simulink model "axi_stream_sobel_filter"  (R2020a)
settings: Solver=VariableStepAuto  StartTime=0.0  StopTime=(height*width)/fs + (width*6)/fs + 128/fs  RelTol=1e-3
PreLoadFcn:
  | clear all;
  | 
  | fs = 100e6;
PostLoadFcn:
  | ratio = 1/6;
  | set(0,'units','pixels');
  | pixels = get(0,'screensize');
  | point1 = round(pixels(3)*ratio);
  | point2 = round(pixels(4)*ratio);
  | point3 = pixels(3)-round(pixels(3)*ratio);
  | point4 = pixels(4)-round(pixels(4)*ratio);
  | h = get_param(gcs,'handle');
  | set_param(h,'location',[point1 point2 point3 point4]);
  | pause(0.2);
  | set_param(h,'Zoomfactor','fit to view');
  | 
  | clear ratio pixels point1 point2 point3 point4 h
  | 
  | % https://uk.mathworks.com/matlabcentral/answers/358413-open-simulink-model-with-set-window-size-and-position
InitFcn:
  | height = str2num(get_param([bdroot, '/Image Properties'], 'height'));
  | width = str2num(get_param([bdroot, '/Image Properties'], 'width'));
  | I = imresize(eval(get_param([bdroot, '/Image Properties'], 'image')), [(height) (width)]);
  | I = padarray(I, [1 1], 'replicate');
  | bufferOut = uint32(double(I(:,:,1))*2^16 + double(I(:,:,3))*2^8 + double(I(:,:,2)));
  | bufferOut = reshape(bufferOut', [width+2, height+2]);
  | bufferOut = bufferOut(:);
StopFcn:
  | imtool(I);
  | imtool(uint8(reshape(bufferIn, [width, height])'));
undefined symbols (not defined in the file): AXI4, Lite
libraries: xbsIndex_r4 x131, hdlsllib x3, dspsrcs4 x2, simulink x1
(part 2 of 2)

== system axi_stream_sobel_filter/DUT/Algorithm/Sobel Edge Filter/Thresholding ==
  Threshold : Inport
  Gmag : Inport  Port=2
  Constant : xbsIndex_r4/Constant  const=255  gui_display_data_type=Fixed-point  arith_type=Unsigned  n_bits=8  bin_pt=0  preci_type=Single  exp_width=8  frac_width=24  explicit_period=on  period=1/100e6  equ=P=C  opselect=C  inp2=PCIN>>17  opr=+  inp1=P  carry=CIN  dbl_ovrd=off  block_type=constant
  Constant1 : xbsIndex_r4/Constant  const=0  gui_display_data_type=Fixed-point  arith_type=Unsigned  n_bits=8  bin_pt=0  preci_type=Single  exp_width=8  frac_width=24  explicit_period=on  period=1/100e6  equ=P=C  opselect=C  inp2=PCIN>>17  opr=+  inp1=P  carry=CIN  dbl_ovrd=off  block_type=constant
  Mux : xbsIndex_r4/Mux  inputs=2  en=off  latency=1  precision=Full  arith_type=Unsigned  n_bits=16  bin_pt=14  quantization=Truncate  overflow=Wrap  dbl_ovrd=off  block_type=mux
  Relational : xbsIndex_r4/Relational  mode=a>=b  op_type=Bool  en=off  latency=0  dbl_ovrd=off  block_type=relational
  Edge : Outport  VectorParamsAs1DForOutWhenUnconnected=off
  wires:
  Threshold/1 -> Relational/2
  Relational/1 -> Mux/1
  Constant/1 -> Mux/3
  Constant1/1 -> Mux/2
  Gmag/1 -> Relational/1
  Mux/1 -> Edge/1

== system axi_stream_sobel_filter/DUT/Algorithm/Sobel Edge Filter/Filter Function/Gx Operation ==
  w00 : Inport
  w02 : Inport  Port=2
  w10 : Inport  Port=3
  w12 : Inport  Port=4
  w20 : Inport  Port=5
  w22 : Inport  Port=6
  AddSub : xbsIndex_r4/AddSub  mode=Subtraction  use_carryin=off  use_carryout=off  en=off  latency=1  precision=Full  arith_type=Unsigned  n_bits=16  bin_pt=14  quantization=Truncate  overflow=Wrap  use_behavioral_HDL=off  hw_selection=Fabric  pipelined=off  dbl_ovrd=off  block_type=addsub
  AddSub1 : xbsIndex_r4/AddSub  mode=Subtraction  use_carryin=off  use_carryout=off  en=off  latency=1  precision=Full  arith_type=Unsigned  n_bits=16  bin_pt=14  quantization=Truncate  overflow=Wrap  use_behavioral_HDL=off  hw_selection=Fabric  pipelined=off  dbl_ovrd=off  block_type=addsub
  AddSub2 : xbsIndex_r4/AddSub  mode=Subtraction  use_carryin=off  use_carryout=off  en=off  latency=1  precision=Full  arith_type=Unsigned  n_bits=16  bin_pt=14  quantization=Truncate  overflow=Wrap  use_behavioral_HDL=off  hw_selection=Fabric  pipelined=off  dbl_ovrd=off  block_type=addsub
  AddSub3 : xbsIndex_r4/AddSub  mode=Addition  use_carryin=off  use_carryout=off  en=off  latency=1  precision=Full  arith_type=Unsigned  n_bits=16  bin_pt=14  quantization=Truncate  overflow=Wrap  use_behavioral_HDL=off  hw_selection=Fabric  pipelined=off  dbl_ovrd=off  block_type=addsub
  AddSub4 : xbsIndex_r4/AddSub  mode=Addition  use_carryin=off  use_carryout=off  en=off  latency=1  precision=Full  arith_type=Unsigned  n_bits=16  bin_pt=14  quantization=Truncate  overflow=Wrap  use_behavioral_HDL=off  hw_selection=Fabric  pipelined=off  dbl_ovrd=off  block_type=addsub
  CMult : xbsIndex_r4/CMult  const=2  gui_display_data_type=Fixed-point  const_n_bits=2  const_bin_pt=0  float_type=Single  exp_bits=8  fraction_bits=24  en=off  latency=1  precision=Full  arith_type="Signed  (2's comp)"  n_bits=16  bin_pt=14  quantization=Truncate  overflow=Wrap  use_behavioral_HDL=off  mem_type=Distributed RAM  pipeline=off  dbl_ovrd=off  block_type=cmult
  CMult1 : xbsIndex_r4/CMult  const=2  gui_display_data_type=Fixed-point  const_n_bits=2  const_bin_pt=0  float_type=Single  exp_bits=8  fraction_bits=24  en=off  latency=1  precision=Full  arith_type="Signed  (2's comp)"  n_bits=16  bin_pt=14  quantization=Truncate  overflow=Wrap  use_behavioral_HDL=off  mem_type=Distributed RAM  pipeline=off  dbl_ovrd=off  block_type=cmult
  Gx : Outport  VectorParamsAs1DForOutWhenUnconnected=off
  wires:
  AddSub4/1 -> Gx/1
  AddSub1/1 -> AddSub4/2
  AddSub3/1 -> AddSub4/1
  AddSub2/1 -> AddSub3/2
  w20/1 -> AddSub2/2
  w22/1 -> AddSub2/1
  AddSub/1 -> AddSub3/1
  CMult/1 -> AddSub1/2
  CMult1/1 -> AddSub1/1
  w12/1 -> CMult1/1
  w10/1 -> CMult/1
  w00/1 -> AddSub/2
  w02/1 -> AddSub/1

== system axi_stream_sobel_filter/DUT/Algorithm/Sobel Edge Filter/Filter Function/Gy Operation ==
  w00 : Inport
  w01 : Inport  Port=2
  w02 : Inport  Port=3
  w20 : Inport  Port=4
  w21 : Inport  Port=5
  w22 : Inport  Port=6
  AddSub : xbsIndex_r4/AddSub  mode=Subtraction  use_carryin=off  use_carryout=off  en=off  latency=1  precision=Full  arith_type=Unsigned  n_bits=16  bin_pt=14  quantization=Truncate  overflow=Wrap  use_behavioral_HDL=off  hw_selection=Fabric  pipelined=off  dbl_ovrd=off  block_type=addsub
  AddSub1 : xbsIndex_r4/AddSub  mode=Subtraction  use_carryin=off  use_carryout=off  en=off  latency=1  precision=Full  arith_type=Unsigned  n_bits=16  bin_pt=14  quantization=Truncate  overflow=Wrap  use_behavioral_HDL=off  hw_selection=Fabric  pipelined=off  dbl_ovrd=off  block_type=addsub
  AddSub2 : xbsIndex_r4/AddSub  mode=Subtraction  use_carryin=off  use_carryout=off  en=off  latency=1  precision=Full  arith_type=Unsigned  n_bits=16  bin_pt=14  quantization=Truncate  overflow=Wrap  use_behavioral_HDL=off  hw_selection=Fabric  pipelined=off  dbl_ovrd=off  block_type=addsub
  AddSub3 : xbsIndex_r4/AddSub  mode=Addition  use_carryin=off  use_carryout=off  en=off  latency=1  precision=Full  arith_type=Unsigned  n_bits=16  bin_pt=14  quantization=Truncate  overflow=Wrap  use_behavioral_HDL=off  hw_selection=Fabric  pipelined=off  dbl_ovrd=off  block_type=addsub
  AddSub4 : xbsIndex_r4/AddSub  mode=Addition  use_carryin=off  use_carryout=off  en=off  latency=1  precision=Full  arith_type=Unsigned  n_bits=16  bin_pt=14  quantization=Truncate  overflow=Wrap  use_behavioral_HDL=off  hw_selection=Fabric  pipelined=off  dbl_ovrd=off  block_type=addsub
  CMult : xbsIndex_r4/CMult  const=2  gui_display_data_type=Fixed-point  const_n_bits=2  const_bin_pt=0  float_type=Single  exp_bits=8  fraction_bits=24  en=off  latency=1  precision=Full  arith_type="Signed  (2's comp)"  n_bits=16  bin_pt=14  quantization=Truncate  overflow=Wrap  use_behavioral_HDL=off  mem_type=Distributed RAM  pipeline=off  dbl_ovrd=off  block_type=cmult
  CMult1 : xbsIndex_r4/CMult  const=2  gui_display_data_type=Fixed-point  const_n_bits=2  const_bin_pt=0  float_type=Single  exp_bits=8  fraction_bits=24  en=off  latency=1  precision=Full  arith_type="Signed  (2's comp)"  n_bits=16  bin_pt=14  quantization=Truncate  overflow=Wrap  use_behavioral_HDL=off  mem_type=Distributed RAM  pipeline=off  dbl_ovrd=off  block_type=cmult
  Gy : Outport  VectorParamsAs1DForOutWhenUnconnected=off
  wires:
  w02/1 -> AddSub2/2
  CMult1/1 -> AddSub1/1
  CMult/1 -> AddSub1/2
  AddSub/1 -> AddSub3/1
  w22/1 -> AddSub2/1
  AddSub2/1 -> AddSub3/2
  AddSub3/1 -> AddSub4/1
  AddSub1/1 -> AddSub4/2
  w20/1 -> AddSub/1
  w00/1 -> AddSub/2
  w01/1 -> CMult/1
  AddSub4/1 -> Gy/1
  w21/1 -> CMult1/1
